simulink model "c2_5jiangweiguanceqi"  (R2019b)
settings: Solver=VariableStepAuto  StartTime=0.0  StopTime=50  RelTol=1e-3  EnableMultiTasking=on
settings Model: Creator=dell  LastModifiedBy=wy151
settings DataIOCC: LimitDataPoints=on  ReturnWorkspaceOutputs=off
settings OptimizationCC: LifeSpan=inf
settings DebuggingCC: AllowSymbolicDim=off  SFUnexpectedBacktrackingDiag=warning  SFNoUnconditionalDefaultTransitionDiag=warning  SFExecutionAtInitializationDiag=none  ArithmeticOperatorsInVariantConditions=warning
settings ModelReferenceCC: PropagateSignalLabelsOutOfModel=off
settings SFSimCC: SimUseLocalCustomCode=off  CustomCodeUndefinedFunction=UseInterfaceOnly
settings RTWCC: RTWUseLocalCustomCode=off
settings CodeAppCC: StateflowObjectComments=on
settings GRTTargetCC: TargetLangStandard=C89/C90 (ANSI)
settings ConfigComp: CovMetricSettings=dw  CovHtmlReporting=on  CovSaveCumulativeToWorkspaceVar=on  CovSaveSingleToWorkspaceVar=on  CovExternalEMLEnable=off

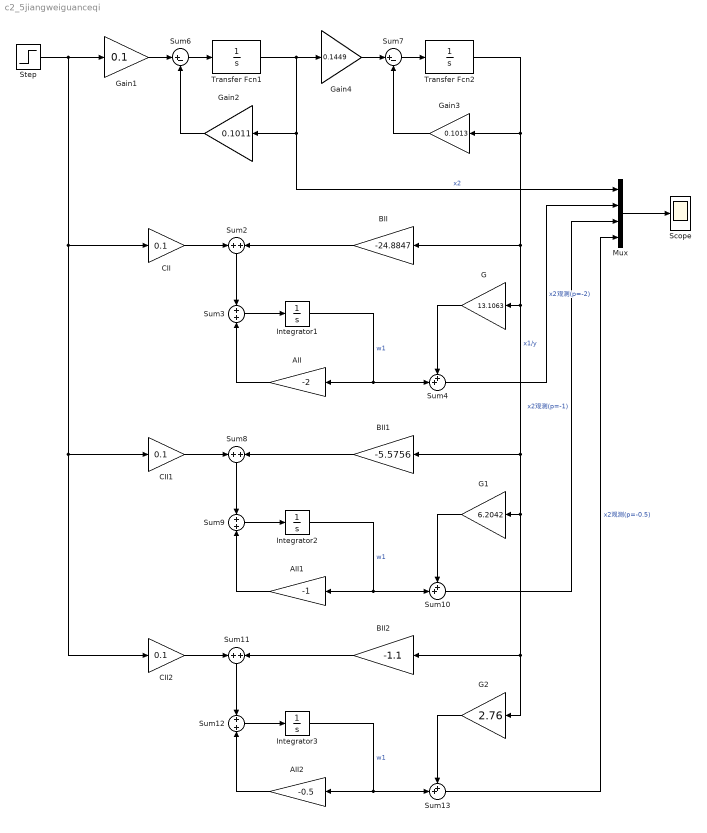
== system c2_5jiangweiguanceqi ==
  AII : Gain  Gain=-2
  AII1 : Gain  Gain=-1
  AII2 : Gain  Gain=-0.5
  BII : Gain  Gain=-24.8847
  BII1 : Gain  Gain=-5.5756
  BII2 : Gain  Gain=-1.1
  CII : Gain  Gain=0.1
  CII1 : Gain  Gain=0.1
  CII2 : Gain  Gain=0.1
  G : Gain  Gain=13.1063
  G1 : Gain  Gain=6.2042
  G2 : Gain  Gain=2.76
  Gain1 : Gain  Gain=0.1
  Gain2 : Gain  Gain=0.1011
  Gain3 : Gain  Gain=0.1013
  Gain4 : Gain  Gain=0.1449
  Integrator1 : Integrator
  Integrator2 : Integrator
  Integrator3 : Integrator
  Mux : Mux
  Scope : Scope
  Step : Step  SampleTime=0
  Sum10 : Sum  Inputs=++|
  Sum{2..3,8..9,11..12} (6 alike) : Sum  Inputs=+|+
  Sum13 : Sum  Inputs=++|
  Sum4 : Sum  Inputs=++|
  Sum6 : Sum  Inputs=|+-
  Sum7 : Sum  Inputs=|+-
  Transfer Fcn1 : TransferFcn  Denominator=[1 0]
  Transfer Fcn2 : TransferFcn  Denominator=[1 0]
  wires:
  Transfer Fcn1/1 -> Gain2/1, Mux/1, Gain4/1  "x2"
  Transfer Fcn2/1 -> G1/1, G2/1, BII2/1, BII1/1, G/1, BII/1, Gain3/1  "x1/y"
  CII/1 -> Sum2/1
  BII/1 -> Sum2/2
  Sum3/1 -> Integrator1/1
  Integrator1/1 -> Sum4/2, AII/1  "w1"
  AII/1 -> Sum3/2
  G/1 -> Sum4/1
  Mux/1 -> Scope/1
  Step/1 -> CII/1, CII1/1, CII2/1, Gain1/1
  Sum2/1 -> Sum3/1
  Gain2/1 -> Sum6/2
  Gain1/1 -> Sum6/1
  Sum6/1 -> Transfer Fcn1/1
  Gain4/1 -> Sum7/1
  Gain3/1 -> Sum7/2
  Sum7/1 -> Transfer Fcn2/1
  BII1/1 -> Sum8/2
  Sum9/1 -> Integrator2/1
  Sum8/1 -> Sum9/1
  G1/1 -> Sum10/1
  AII1/1 -> Sum9/2
  Integrator2/1 -> Sum10/2, AII1/1  "w1"
  CII1/1 -> Sum8/1
  BII2/1 -> Sum11/2
  Sum12/1 -> Integrator3/1
  Sum11/1 -> Sum12/1
  G2/1 -> Sum13/1
  AII2/1 -> Sum12/2
  Integrator3/1 -> Sum13/2, AII2/1  "w1"
  CII2/1 -> Sum11/1
  Sum13/1 -> Mux/4  "x2观测(p=-0.5)"
  Sum4/1 -> Mux/2  "x2观测(p=-2)"
  Sum10/1 -> Mux/3  "x2观测(p=-1)"
